simulink model "ckt1"  (Simulink 7.8)
settings: Solver=ode45  StartTime=0.0  StopTime=10.0  RelTol=1e-3
libraries: fuzblock x17
settings Model: Creator=Administrator  LastModifiedBy=Acer
settings DebuggingCC: FcnCallInpInsideContextMsg=Use local settings  StrictBusMsg=Warning

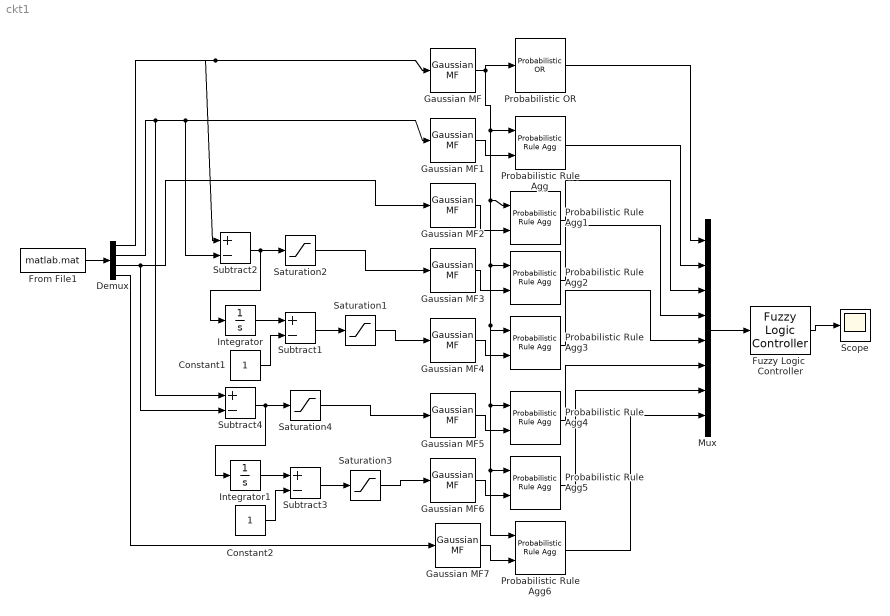
== system ckt1 ==
  Constant1 : Constant
  Constant2 : Constant
  Demux : Demux
  From File1 : FromFile  FileName=matlab.mat  SampleTime=0
  Fuzzy Logic  Controller : fuzblock/Fuzzy Logic  Controller  fis=ashokrules.fis
  Gaussian MF{,1..7} (8 alike) : fuzblock/Membership  Functions/Gaussian MF  sigma=1  mu=0
  Integrator : Integrator
  Integrator1 : Integrator
  Mux : Mux  Inputs=8
  Probabilistic OR : fuzblock/Membership  Functions/Probabilistic OR
  Probabilistic Rule Agg{,1..6} (7 alike) : fuzblock/Membership  Functions/Probabilistic Rule Agg
  Saturation{1..4} (4 alike) : Saturate
  Scope : Scope
  Subtract{1..4} (4 alike) : Sum  Inputs=+-
  wires:
  Gaussian MF/1 -> Probabilistic OR/1, Probabilistic Rule Agg/1, Probabilistic Rule Agg1/1, Probabilistic Rule Agg2/1, Probabilistic Rule Agg3/1, Probabilistic Rule Agg4/1, Probabilistic Rule Agg5/1, Probabilistic Rule Agg6/1
  Gaussian MF1/1 -> Probabilistic Rule Agg/2
  Probabilistic OR/1 -> Mux/1
  Probabilistic Rule Agg/1 -> Mux/2
  Gaussian MF2/1 -> Probabilistic Rule Agg1/2
  Probabilistic Rule Agg1/1 -> Mux/3
  Gaussian MF3/1 -> Probabilistic Rule Agg2/2
  Gaussian MF4/1 -> Probabilistic Rule Agg3/2
  Gaussian MF5/1 -> Probabilistic Rule Agg4/2
  Gaussian MF6/1 -> Probabilistic Rule Agg5/2
  Gaussian MF7/1 -> Probabilistic Rule Agg6/2
  Probabilistic Rule Agg2/1 -> Mux/4
  Probabilistic Rule Agg3/1 -> Mux/5
  Probabilistic Rule Agg4/1 -> Mux/6
  Probabilistic Rule Agg5/1 -> Mux/7
  Probabilistic Rule Agg6/1 -> Mux/8
  Mux/1 -> Fuzzy Logic  Controller/1
  Fuzzy Logic  Controller/1 -> Scope/1
  Integrator/1 -> Subtract1/1
  Constant1/1 -> Subtract1/2
  Subtract1/1 -> Saturation1/1
  Subtract2/1 -> Saturation2/1, Integrator/1
  Saturation2/1 -> Gaussian MF3/1
  Saturation1/1 -> Gaussian MF4/1
  Integrator1/1 -> Subtract3/1
  Constant2/1 -> Subtract3/2
  Subtract3/1 -> Saturation3/1
  Subtract4/1 -> Saturation4/1, Integrator1/1
  Saturation4/1 -> Gaussian MF5/1
  Saturation3/1 -> Gaussian MF6/1
  Demux/1 -> Gaussian MF/1, Subtract2/1
  Demux/2 -> Gaussian MF1/1, Subtract2/2, Subtract4/1
  Demux/3 -> Gaussian MF2/1, Subtract4/2
  Demux/4 -> Gaussian MF7/1
  From File1/1 -> Demux/1
